simulink model "w2_warplab_trigger_proc"  (Simulink 7.7)
settings: Solver=ode45  StartTime=0.0  StopTime=1000  RelTol=1e-3
InitFcn:
  | w2_warplab_trigger_proc_init
StartFcn:
  | w2_warplab_trigger_proc_init
undefined symbols (not defined in the file or in its folder): gcbh, xlBlockLoadCallback, xlGetNormalizedPeriod
libraries: xbsIndex_r4 x819, simulink x1
(part 4 of 6)

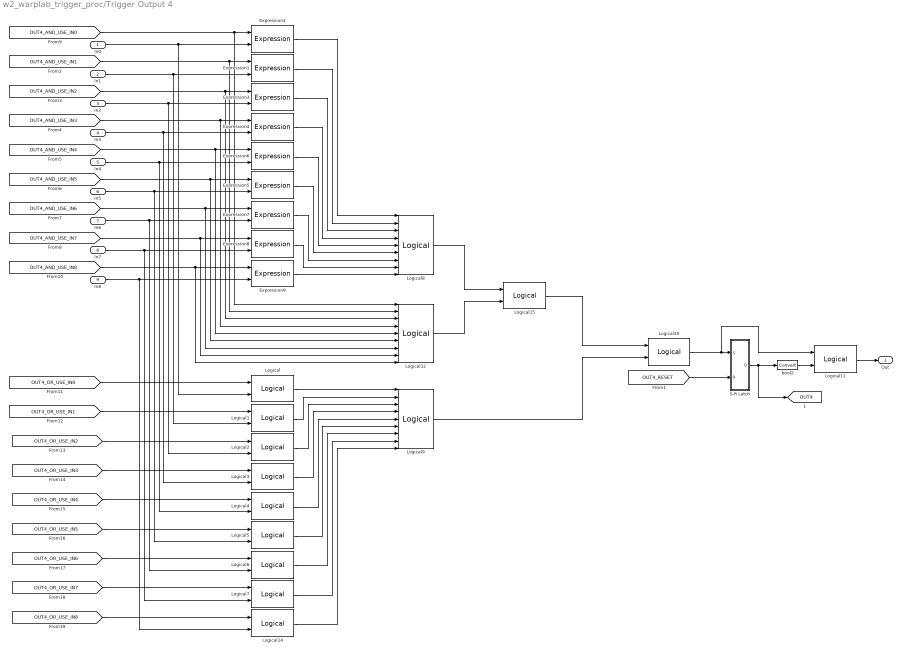
== system w2_warplab_trigger_proc/Trigger Output 4 ==
  In0 : Inport
  In1 : Inport  Port=2
  In2 : Inport  Port=3
  In3 : Inport  Port=4
  In4 : Inport  Port=5
  In5 : Inport  Port=6
  In6 : Inport  Port=7
  In7 : Inport  Port=8
  In8 : Inport  Port=9
  Expression{1..9} (9 alike) : xbsIndex_r4/Expression  expression=~a | (a & b)  align_bp=on  en=off  latency=0  precision=Full  arith_type=Unsigned  n_bits=16  bin_pt=0  dbl_ovrd=off  block_type=expr
  Logical{,1..7,14..15} (10 alike) : xbsIndex_r4/Logical  logical_function=AND  inputs=2  en=off  latency=0  precision=Full  arith_type=Unsigned  n_bits=16  bin_pt=0  align_bp=on  dbl_ovrd=off  block_type=logical
  Logical10 : xbsIndex_r4/Logical  logical_function=OR  inputs=2  en=off  latency=0  precision=Full  arith_type=Unsigned  n_bits=16  bin_pt=0  align_bp=on  dbl_ovrd=off  block_type=logical
  Logical11 : xbsIndex_r4/Logical  logical_function=OR  inputs=2  en=off  latency=0  precision=Full  arith_type=Unsigned  n_bits=16  bin_pt=0  align_bp=on  dbl_ovrd=off  block_type=logical
  Logical12 : xbsIndex_r4/Logical  logical_function=OR  inputs=9  en=off  latency=0  precision=Full  arith_type=Unsigned  n_bits=16  bin_pt=0  align_bp=on  dbl_ovrd=off  block_type=logical
  Logical8 : xbsIndex_r4/Logical  logical_function=AND  inputs=9  en=off  latency=0  precision=Full  arith_type=Unsigned  n_bits=16  bin_pt=0  align_bp=on  dbl_ovrd=off  block_type=logical
  Logical9 : xbsIndex_r4/Logical  logical_function=OR  inputs=9  en=off  latency=0  precision=Full  arith_type=Unsigned  n_bits=16  bin_pt=0  align_bp=on  dbl_ovrd=off  block_type=logical
  S-R Latch : Subsystem
  bool2 : xbsIndex_r4/Convert  gui_display_data_type=Boolean  arith_type=Boolean  n_bits=16  bin_pt=14  float_type=Single  exp_bits=8  fraction_bits=24  quantization=Truncate  overflow=Wrap  en=off  latency=0  dbl_ovrd=off  pipeline=off  block_type=convert
  Out : Outport
  tag scope: OUT4=global
  wires:
  [OUT4_AND_USE_IN0] -> Expression2/1, Logical12/1
  [OUT4_AND_USE_IN1] -> Expression1/1, Logical12/2
  [OUT4_AND_USE_IN2] -> Expression3/1, Logical12/3
  [OUT4_AND_USE_IN3] -> Expression4/1, Logical12/4
  [OUT4_AND_USE_IN4] -> Expression6/1, Logical12/5
  [OUT4_AND_USE_IN5] -> Expression5/1, Logical12/6
  [OUT4_AND_USE_IN6] -> Expression7/1, Logical12/7
  [OUT4_AND_USE_IN7] -> Expression8/1, Logical12/8
  In0/1 -> Logical/2, Expression2/2
  In1/1 -> Expression1/2, Logical1/2
  In2/1 -> Expression3/2, Logical2/2
  In3/1 -> Expression4/2, Logical3/2
  In4/1 -> Expression6/2, Logical4/2
  In5/1 -> Expression5/2, Logical5/2
  In6/1 -> Expression7/2, Logical6/2
  In7/1 -> Expression8/2, Logical7/2
  [OUT4_OR_USE_IN0] -> Logical/1
  [OUT4_OR_USE_IN1] -> Logical1/1
  Expression2/1 -> Logical8/1
  Expression1/1 -> Logical8/2
  Expression3/1 -> Logical8/3
  Expression4/1 -> Logical8/4
  Expression6/1 -> Logical8/5
  Expression5/1 -> Logical8/6
  Expression7/1 -> Logical8/7
  Expression8/1 -> Logical8/8
  Logical/1 -> Logical9/1
  Logical1/1 -> Logical9/2
  Logical2/1 -> Logical9/3
  Logical3/1 -> Logical9/4
  Logical4/1 -> Logical9/5
  Logical5/1 -> Logical9/6
  Logical6/1 -> Logical9/7
  Logical7/1 -> Logical9/8
  Logical9/1 -> Logical10/2
  Logical10/1 -> S-R Latch/1(S), Logical11/1
  [OUT4_RESET] -> S-R Latch/2(R)
  S-R Latch/1(Q) -> [OUT4], bool2/1
  Logical11/1 -> Out/1
  bool2/1 -> Logical11/2
  Logical12/1 -> Logical15/2
  Logical15/1 -> Logical10/1
  [OUT4_AND_USE_IN8] -> Expression9/1, Logical12/9
  In8/1 -> Expression9/2, Logical14/2
  Logical8/1 -> Logical15/1
  Expression9/1 -> Logical8/9
  [OUT4_OR_USE_IN2] -> Logical2/1
  [OUT4_OR_USE_IN3] -> Logical3/1
  [OUT4_OR_USE_IN4] -> Logical4/1
  [OUT4_OR_USE_IN5] -> Logical5/1
  [OUT4_OR_USE_IN6] -> Logical6/1
  [OUT4_OR_USE_IN7] -> Logical7/1
  [OUT4_OR_USE_IN8] -> Logical14/1
  Logical14/1 -> Logical9/9

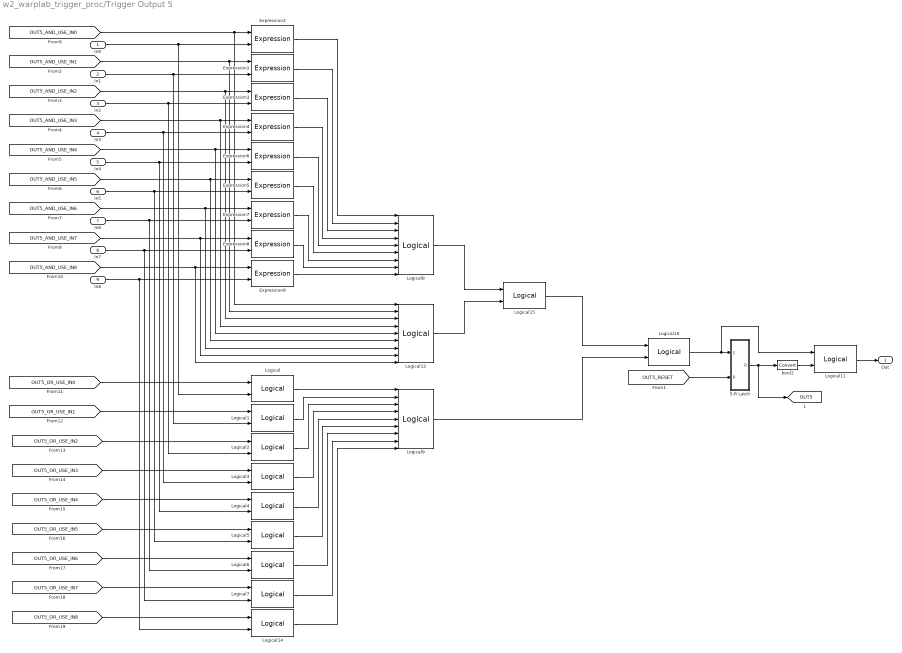
== system w2_warplab_trigger_proc/Trigger Output 5 ==
  In0 : Inport
  In1 : Inport  Port=2
  In2 : Inport  Port=3
  In3 : Inport  Port=4
  In4 : Inport  Port=5
  In5 : Inport  Port=6
  In6 : Inport  Port=7
  In7 : Inport  Port=8
  In8 : Inport  Port=9
  Expression{1..9} (9 alike) : xbsIndex_r4/Expression  expression=~a | (a & b)  align_bp=on  en=off  latency=0  precision=Full  arith_type=Unsigned  n_bits=16  bin_pt=0  dbl_ovrd=off  block_type=expr
  Logical{,1..7,14..15} (10 alike) : xbsIndex_r4/Logical  logical_function=AND  inputs=2  en=off  latency=0  precision=Full  arith_type=Unsigned  n_bits=16  bin_pt=0  align_bp=on  dbl_ovrd=off  block_type=logical
  Logical10 : xbsIndex_r4/Logical  logical_function=OR  inputs=2  en=off  latency=0  precision=Full  arith_type=Unsigned  n_bits=16  bin_pt=0  align_bp=on  dbl_ovrd=off  block_type=logical
  Logical11 : xbsIndex_r4/Logical  logical_function=OR  inputs=2  en=off  latency=0  precision=Full  arith_type=Unsigned  n_bits=16  bin_pt=0  align_bp=on  dbl_ovrd=off  block_type=logical
  Logical12 : xbsIndex_r4/Logical  logical_function=OR  inputs=9  en=off  latency=0  precision=Full  arith_type=Unsigned  n_bits=16  bin_pt=0  align_bp=on  dbl_ovrd=off  block_type=logical
  Logical8 : xbsIndex_r4/Logical  logical_function=AND  inputs=9  en=off  latency=0  precision=Full  arith_type=Unsigned  n_bits=16  bin_pt=0  align_bp=on  dbl_ovrd=off  block_type=logical
  Logical9 : xbsIndex_r4/Logical  logical_function=OR  inputs=9  en=off  latency=0  precision=Full  arith_type=Unsigned  n_bits=16  bin_pt=0  align_bp=on  dbl_ovrd=off  block_type=logical
  S-R Latch : Subsystem
  bool2 : xbsIndex_r4/Convert  gui_display_data_type=Boolean  arith_type=Boolean  n_bits=16  bin_pt=14  float_type=Single  exp_bits=8  fraction_bits=24  quantization=Truncate  overflow=Wrap  en=off  latency=0  dbl_ovrd=off  pipeline=off  block_type=convert
  Out : Outport
  tag scope: OUT5=global
  wires:
  [OUT5_AND_USE_IN0] -> Expression2/1, Logical12/1
  [OUT5_AND_USE_IN1] -> Expression1/1, Logical12/2
  [OUT5_AND_USE_IN2] -> Expression3/1, Logical12/3
  [OUT5_AND_USE_IN3] -> Expression4/1, Logical12/4
  [OUT5_AND_USE_IN4] -> Expression6/1, Logical12/5
  [OUT5_AND_USE_IN5] -> Expression5/1, Logical12/6
  [OUT5_AND_USE_IN6] -> Expression7/1, Logical12/7
  [OUT5_AND_USE_IN7] -> Expression8/1, Logical12/8
  In0/1 -> Logical/2, Expression2/2
  In1/1 -> Expression1/2, Logical1/2
  In2/1 -> Expression3/2, Logical2/2
  In3/1 -> Expression4/2, Logical3/2
  In4/1 -> Expression6/2, Logical4/2
  In5/1 -> Expression5/2, Logical5/2
  In6/1 -> Expression7/2, Logical6/2
  In7/1 -> Expression8/2, Logical7/2
  [OUT5_OR_USE_IN0] -> Logical/1
  [OUT5_OR_USE_IN1] -> Logical1/1
  Expression2/1 -> Logical8/1
  Expression1/1 -> Logical8/2
  Expression3/1 -> Logical8/3
  Expression4/1 -> Logical8/4
  Expression6/1 -> Logical8/5
  Expression5/1 -> Logical8/6
  Expression7/1 -> Logical8/7
  Expression8/1 -> Logical8/8
  Logical/1 -> Logical9/1
  Logical1/1 -> Logical9/2
  Logical2/1 -> Logical9/3
  Logical3/1 -> Logical9/4
  Logical4/1 -> Logical9/5
  Logical5/1 -> Logical9/6
  Logical6/1 -> Logical9/7
  Logical7/1 -> Logical9/8
  Logical9/1 -> Logical10/2
  Logical10/1 -> S-R Latch/1(S), Logical11/1
  [OUT5_RESET] -> S-R Latch/2(R)
  S-R Latch/1(Q) -> [OUT5], bool2/1
  Logical11/1 -> Out/1
  bool2/1 -> Logical11/2
  Logical12/1 -> Logical15/2
  Logical15/1 -> Logical10/1
  [OUT5_AND_USE_IN8] -> Expression9/1, Logical12/9
  In8/1 -> Expression9/2, Logical14/2
  Logical8/1 -> Logical15/1
  Expression9/1 -> Logical8/9
  [OUT5_OR_USE_IN2] -> Logical2/1
  [OUT5_OR_USE_IN3] -> Logical3/1
  [OUT5_OR_USE_IN4] -> Logical4/1
  [OUT5_OR_USE_IN5] -> Logical5/1
  [OUT5_OR_USE_IN6] -> Logical6/1
  [OUT5_OR_USE_IN7] -> Logical7/1
  [OUT5_OR_USE_IN8] -> Logical14/1
  Logical14/1 -> Logical9/9

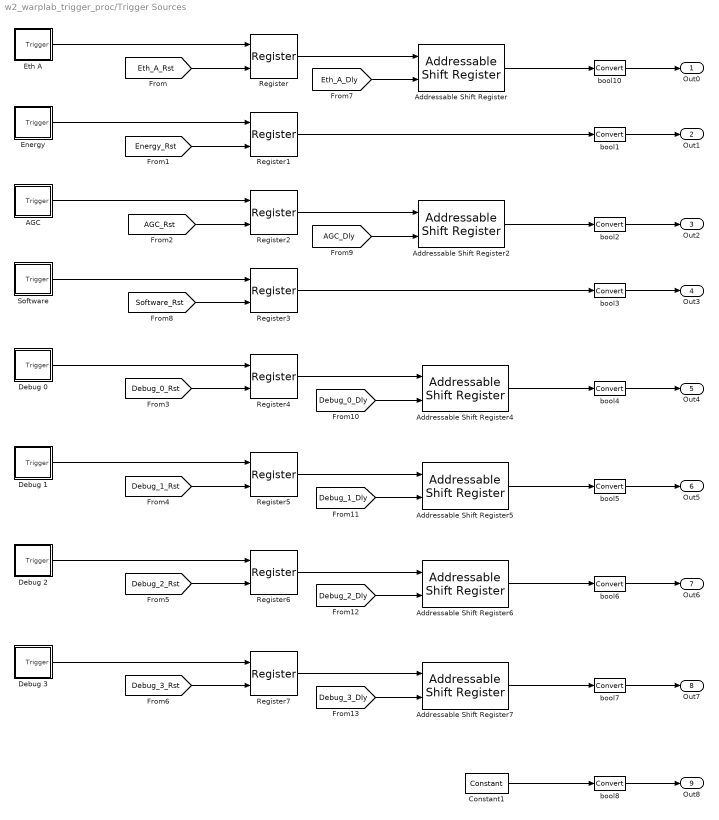
== system w2_warplab_trigger_proc/Trigger Sources ==
  AGC : Subsystem
  Addressable Shift Register{,2,4..7} (6 alike) : xbsIndex_r4/Addressable Shift Register  infer_latency=off  depth=32  initVector=[0]  en=off  dbl_ovrd=off  use_behavioral_HDL=off  Optimization=Resource  block_type=addrsr
      settings: infoedit="Delay of configurable length.  Any element in the delay line can be addressed and driven onto the output port.<br><br>Hardware notes: This block is implemented using SRL16s. If Virtex-4 or Spartan-3 device is used, multiple SRLC16s are cascaded together."
  Constant1 : xbsIndex_r4/Constant  const=0  gui_display_data_type=Fixed-point  arith_type=Unsigned  n_bits=1  bin_pt=0  preci_type=Single  exp_width=8  frac_width=24  explicit_period=off  period=1  equ=P=C  opselect=C  inp2=PCIN>>17  opr=+  inp1=P  carry=CIN  dbl_ovrd=off  block_type=constant
  Debug 0 : Subsystem
  Debug 1 : Subsystem
  Debug 2 : Subsystem
  Debug 3 : Subsystem
  Energy : Subsystem
  Eth A : Subsystem
  Register{,1..7} (8 alike) : xbsIndex_r4/Register  init=0  rst=on  en=off  dbl_ovrd=off  block_type=register
  Software : Subsystem
  bool{1..8,10} (9 alike) : xbsIndex_r4/Convert  gui_display_data_type=Boolean  arith_type=Boolean  n_bits=16  bin_pt=14  float_type=Single  exp_bits=8  fraction_bits=24  quantization=Truncate  overflow=Wrap  en=off  latency=0  dbl_ovrd=off  pipeline=off  block_type=convert
  Out0 : Outport
  Out1 : Outport  Port=2
  Out2 : Outport  Port=3
  Out3 : Outport  Port=4
  Out4 : Outport  Port=5
  Out5 : Outport  Port=6
  Out6 : Outport  Port=7
  Out7 : Outport  Port=8
  Out8 : Outport  Port=9
  wires:
  Energy/1(Trigger) -> Register1/1
  [Energy_Rst] -> Register1/2
  AGC/1(Trigger) -> Register2/1
  [AGC_Rst] -> Register2/2
  [Debug_0_Rst] -> Register4/2
  [Debug_1_Rst] -> Register5/2
  [Debug_2_Rst] -> Register6/2
  [Debug_3_Rst] -> Register7/2
  [Debug_0_Dly] -> Addressable Shift Register4/2
  Register4/1 -> Addressable Shift Register4/1
  [Debug_1_Dly] -> Addressable Shift Register5/2
  Register5/1 -> Addressable Shift Register5/1
  [Debug_2_Dly] -> Addressable Shift Register6/2
  Register6/1 -> Addressable Shift Register6/1
  [Debug_3_Dly] -> Addressable Shift Register7/2
  Register7/1 -> Addressable Shift Register7/1
  Software/1(Trigger) -> Register3/1
  [Software_Rst] -> Register3/2
  Register1/1 -> bool1/1
  Register3/1 -> bool3/1
  Addressable Shift Register4/1 -> bool4/1
  Addressable Shift Register5/1 -> bool5/1
  Addressable Shift Register6/1 -> bool6/1
  Addressable Shift Register7/1 -> bool7/1
  bool10/1 -> Out0/1
  bool1/1 -> Out1/1
  bool2/1 -> Out2/1
  bool3/1 -> Out3/1
  bool4/1 -> Out4/1
  bool5/1 -> Out5/1
  bool6/1 -> Out6/1
  bool7/1 -> Out7/1
  [AGC_Dly] -> Addressable Shift Register2/2
  Register2/1 -> Addressable Shift Register2/1
  Addressable Shift Register2/1 -> bool2/1
  bool8/1 -> Out8/1
  Debug 0/1(Trigger) -> Register4/1
  Debug 1/1(Trigger) -> Register5/1
  Debug 2/1(Trigger) -> Register6/1
  Debug 3/1(Trigger) -> Register7/1
  Constant1/1 -> bool8/1
  Eth A/1(Trigger) -> Register/1
  [Eth_A_Rst] -> Register/2
  Register/1 -> Addressable Shift Register/1
  [Eth_A_Dly] -> Addressable Shift Register/2
  Addressable Shift Register/1 -> bool10/1

== system w2_warplab_trigger_proc/Registers/Input Configuration Slice0 ==
  32b : Inport
  b29 : xbsIndex_r4/Slice  nbits=1  boolean_output=off  mode=Lower Bit Location + Width  bit1=0  base1=MSB of Input  bit0=29  base0=LSB of Input  dbl_ovrd=off  block_type=slice
  b30 : xbsIndex_r4/Slice  nbits=1  boolean_output=off  mode=Lower Bit Location + Width  bit1=0  base1=MSB of Input  bit0=30  base0=LSB of Input  dbl_ovrd=off  block_type=slice
  b31 : xbsIndex_r4/Slice  nbits=1  boolean_output=off  mode=Lower Bit Location + Width  bit1=0  base1=MSB of Input  bit0=31  base0=LSB of Input  dbl_ovrd=off  block_type=slice
  b[0:4] : xbsIndex_r4/Slice  nbits=5  boolean_output=off  mode=Lower Bit Location + Width  bit1=0  base1=MSB of Input  bit0=0  base0=LSB of Input  dbl_ovrd=off  block_type=slice
  Delay : Outport
  HW_SW_Sel : Outport  Port=2
  Debounce : Outport  Port=3
  Reset : Outport  Port=4
  wires:
  b31/1 -> Reset/1
  b30/1 -> Debounce/1
  b[0:4]/1 -> Delay/1
  32b/1 -> b[0:4]/1, b30/1, b31/1, b29/1
  b29/1 -> HW_SW_Sel/1

== system w2_warplab_trigger_proc/Registers/Input Configuration Slice1 ==
  32b : Inport
  b30 : xbsIndex_r4/Slice  nbits=1  boolean_output=off  mode=Lower Bit Location + Width  bit1=0  base1=MSB of Input  bit0=30  base0=LSB of Input  dbl_ovrd=off  block_type=slice
  b31 : xbsIndex_r4/Slice  nbits=1  boolean_output=off  mode=Lower Bit Location + Width  bit1=0  base1=MSB of Input  bit0=31  base0=LSB of Input  dbl_ovrd=off  block_type=slice
  b[0:4] : xbsIndex_r4/Slice  nbits=5  boolean_output=off  mode=Lower Bit Location + Width  bit1=0  base1=MSB of Input  bit0=0  base0=LSB of Input  dbl_ovrd=off  block_type=slice
  Delay : Outport
  Debounce : Outport  Port=2
  Reset : Outport  Port=3
  wires:
  b31/1 -> Reset/1
  b30/1 -> Debounce/1
  b[0:4]/1 -> Delay/1
  32b/1 -> b[0:4]/1, b30/1, b31/1

== system w2_warplab_trigger_proc/Registers/Input Configuration Slice2 ==
  32b : Inport
  b30 : xbsIndex_r4/Slice  nbits=1  boolean_output=off  mode=Lower Bit Location + Width  bit1=0  base1=MSB of Input  bit0=30  base0=LSB of Input  dbl_ovrd=off  block_type=slice
  b31 : xbsIndex_r4/Slice  nbits=1  boolean_output=off  mode=Lower Bit Location + Width  bit1=0  base1=MSB of Input  bit0=31  base0=LSB of Input  dbl_ovrd=off  block_type=slice
  b[0:4] : xbsIndex_r4/Slice  nbits=5  boolean_output=off  mode=Lower Bit Location + Width  bit1=0  base1=MSB of Input  bit0=0  base0=LSB of Input  dbl_ovrd=off  block_type=slice
  Delay : Outport
  Debounce : Outport  Port=2
  Reset : Outport  Port=3
  wires:
  b31/1 -> Reset/1
  b30/1 -> Debounce/1
  b[0:4]/1 -> Delay/1
  32b/1 -> b[0:4]/1, b30/1, b31/1

== system w2_warplab_trigger_proc/Registers/Input Configuration Slice3 ==
  32b : Inport
  b30 : xbsIndex_r4/Slice  nbits=1  boolean_output=off  mode=Lower Bit Location + Width  bit1=0  base1=MSB of Input  bit0=30  base0=LSB of Input  dbl_ovrd=off  block_type=slice
  b31 : xbsIndex_r4/Slice  nbits=1  boolean_output=off  mode=Lower Bit Location + Width  bit1=0  base1=MSB of Input  bit0=31  base0=LSB of Input  dbl_ovrd=off  block_type=slice
  b[0:4] : xbsIndex_r4/Slice  nbits=5  boolean_output=off  mode=Lower Bit Location + Width  bit1=0  base1=MSB of Input  bit0=0  base0=LSB of Input  dbl_ovrd=off  block_type=slice
  Delay : Outport
  Debounce : Outport  Port=2
  Reset : Outport  Port=3
  wires:
  b31/1 -> Reset/1
  b30/1 -> Debounce/1
  b[0:4]/1 -> Delay/1
  32b/1 -> b[0:4]/1, b30/1, b31/1

== system w2_warplab_trigger_proc/Registers/Input Configuration Slice4 ==
  32b : Inport
  b30 : xbsIndex_r4/Slice  nbits=1  boolean_output=off  mode=Lower Bit Location + Width  bit1=0  base1=MSB of Input  bit0=30  base0=LSB of Input  dbl_ovrd=off  block_type=slice
  b31 : xbsIndex_r4/Slice  nbits=1  boolean_output=off  mode=Lower Bit Location + Width  bit1=0  base1=MSB of Input  bit0=31  base0=LSB of Input  dbl_ovrd=off  block_type=slice
  b[0:4] : xbsIndex_r4/Slice  nbits=5  boolean_output=off  mode=Lower Bit Location + Width  bit1=0  base1=MSB of Input  bit0=0  base0=LSB of Input  dbl_ovrd=off  block_type=slice
  Delay : Outport
  Debounce : Outport  Port=2
  Reset : Outport  Port=3
  wires:
  b31/1 -> Reset/1
  b30/1 -> Debounce/1
  b[0:4]/1 -> Delay/1
  32b/1 -> b[0:4]/1, b30/1, b31/1

== system w2_warplab_trigger_proc/Registers/Input Configuration Slice5 ==
  32b : Inport
  b30 : xbsIndex_r4/Slice  nbits=1  boolean_output=off  mode=Lower Bit Location + Width  bit1=0  base1=MSB of Input  bit0=30  base0=LSB of Input  dbl_ovrd=off  block_type=slice
  b31 : xbsIndex_r4/Slice  nbits=1  boolean_output=off  mode=Lower Bit Location + Width  bit1=0  base1=MSB of Input  bit0=31  base0=LSB of Input  dbl_ovrd=off  block_type=slice
  b[0:4] : xbsIndex_r4/Slice  nbits=5  boolean_output=off  mode=Lower Bit Location + Width  bit1=0  base1=MSB of Input  bit0=0  base0=LSB of Input  dbl_ovrd=off  block_type=slice
  Delay : Outport
  Debounce : Outport  Port=2
  Reset : Outport  Port=3
  wires:
  b31/1 -> Reset/1
  b30/1 -> Debounce/1
  b[0:4]/1 -> Delay/1
  32b/1 -> b[0:4]/1, b30/1, b31/1

== system w2_warplab_trigger_proc/Registers/Input Configuration Slice6 ==
  32b : Inport
  b30 : xbsIndex_r4/Slice  nbits=1  boolean_output=off  mode=Lower Bit Location + Width  bit1=0  base1=MSB of Input  bit0=30  base0=LSB of Input  dbl_ovrd=off  block_type=slice
  b31 : xbsIndex_r4/Slice  nbits=1  boolean_output=off  mode=Lower Bit Location + Width  bit1=0  base1=MSB of Input  bit0=31  base0=LSB of Input  dbl_ovrd=off  block_type=slice
  b[0:4] : xbsIndex_r4/Slice  nbits=5  boolean_output=off  mode=Lower Bit Location + Width  bit1=0  base1=MSB of Input  bit0=0  base0=LSB of Input  dbl_ovrd=off  block_type=slice
  Delay : Outport
  Debounce : Outport  Port=2
  Reset : Outport  Port=3
  wires:
  b31/1 -> Reset/1
  b30/1 -> Debounce/1
  b[0:4]/1 -> Delay/1
  32b/1 -> b[0:4]/1, b30/1, b31/1

== system w2_warplab_trigger_proc/Registers/Input Configuration Slice7 ==
  32b : Inport
  b30 : xbsIndex_r4/Slice  nbits=1  boolean_output=off  mode=Lower Bit Location + Width  bit1=0  base1=MSB of Input  bit0=30  base0=LSB of Input  dbl_ovrd=off  block_type=slice
  b31 : xbsIndex_r4/Slice  nbits=1  boolean_output=off  mode=Lower Bit Location + Width  bit1=0  base1=MSB of Input  bit0=31  base0=LSB of Input  dbl_ovrd=off  block_type=slice
  b[0:4] : xbsIndex_r4/Slice  nbits=5  boolean_output=off  mode=Lower Bit Location + Width  bit1=0  base1=MSB of Input  bit0=0  base0=LSB of Input  dbl_ovrd=off  block_type=slice
  Delay : Outport
  Debounce : Outport  Port=2
  Reset : Outport  Port=3
  wires:
  b31/1 -> Reset/1
  b30/1 -> Debounce/1
  b[0:4]/1 -> Delay/1
  32b/1 -> b[0:4]/1, b30/1, b31/1

== system w2_warplab_trigger_proc/Registers/Input Configuration Slice8 ==
  32b : Inport
  b29 : xbsIndex_r4/Slice  nbits=1  boolean_output=off  mode=Lower Bit Location + Width  bit1=0  base1=MSB of Input  bit0=29  base0=LSB of Input  dbl_ovrd=off  block_type=slice
  b30 : xbsIndex_r4/Slice  nbits=1  boolean_output=off  mode=Lower Bit Location + Width  bit1=0  base1=MSB of Input  bit0=30  base0=LSB of Input  dbl_ovrd=off  block_type=slice
  b31 : xbsIndex_r4/Slice  nbits=1  boolean_output=off  mode=Lower Bit Location + Width  bit1=0  base1=MSB of Input  bit0=31  base0=LSB of Input  dbl_ovrd=off  block_type=slice
  b[0:4] : xbsIndex_r4/Slice  nbits=5  boolean_output=off  mode=Lower Bit Location + Width  bit1=0  base1=MSB of Input  bit0=0  base0=LSB of Input  dbl_ovrd=off  block_type=slice
  Delay : Outport
  HW_SW_Sel : Outport  Port=2
  Debounce : Outport  Port=3
  Reset : Outport  Port=4
  wires:
  b31/1 -> Reset/1
  b30/1 -> Debounce/1
  b[0:4]/1 -> Delay/1
  32b/1 -> b[0:4]/1, b30/1, b31/1, b29/1
  b29/1 -> HW_SW_Sel/1

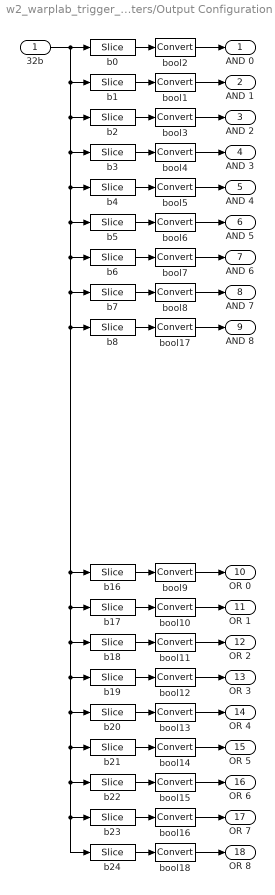
== system w2_warplab_trigger_proc/Registers/Output Configuration Slice ==
  32b : Inport
  b0 : xbsIndex_r4/Slice  nbits=1  boolean_output=off  mode=Lower Bit Location + Width  bit1=0  base1=MSB of Input  bit0=0  base0=LSB of Input  dbl_ovrd=off  block_type=slice
  b1 : xbsIndex_r4/Slice  nbits=1  boolean_output=off  mode=Lower Bit Location + Width  bit1=0  base1=MSB of Input  bit0=1  base0=LSB of Input  dbl_ovrd=off  block_type=slice
  b16 : xbsIndex_r4/Slice  nbits=1  boolean_output=off  mode=Lower Bit Location + Width  bit1=0  base1=MSB of Input  bit0=16  base0=LSB of Input  dbl_ovrd=off  block_type=slice
  b17 : xbsIndex_r4/Slice  nbits=1  boolean_output=off  mode=Lower Bit Location + Width  bit1=0  base1=MSB of Input  bit0=17  base0=LSB of Input  dbl_ovrd=off  block_type=slice
  b18 : xbsIndex_r4/Slice  nbits=1  boolean_output=off  mode=Lower Bit Location + Width  bit1=0  base1=MSB of Input  bit0=18  base0=LSB of Input  dbl_ovrd=off  block_type=slice
  b19 : xbsIndex_r4/Slice  nbits=1  boolean_output=off  mode=Lower Bit Location + Width  bit1=0  base1=MSB of Input  bit0=19  base0=LSB of Input  dbl_ovrd=off  block_type=slice
  b2 : xbsIndex_r4/Slice  nbits=1  boolean_output=off  mode=Lower Bit Location + Width  bit1=0  base1=MSB of Input  bit0=2  base0=LSB of Input  dbl_ovrd=off  block_type=slice
  b20 : xbsIndex_r4/Slice  nbits=1  boolean_output=off  mode=Lower Bit Location + Width  bit1=0  base1=MSB of Input  bit0=20  base0=LSB of Input  dbl_ovrd=off  block_type=slice
  b21 : xbsIndex_r4/Slice  nbits=1  boolean_output=off  mode=Lower Bit Location + Width  bit1=0  base1=MSB of Input  bit0=21  base0=LSB of Input  dbl_ovrd=off  block_type=slice
  b22 : xbsIndex_r4/Slice  nbits=1  boolean_output=off  mode=Lower Bit Location + Width  bit1=0  base1=MSB of Input  bit0=22  base0=LSB of Input  dbl_ovrd=off  block_type=slice
  b23 : xbsIndex_r4/Slice  nbits=1  boolean_output=off  mode=Lower Bit Location + Width  bit1=0  base1=MSB of Input  bit0=23  base0=LSB of Input  dbl_ovrd=off  block_type=slice
  b24 : xbsIndex_r4/Slice  nbits=1  boolean_output=off  mode=Lower Bit Location + Width  bit1=0  base1=MSB of Input  bit0=24  base0=LSB of Input  dbl_ovrd=off  block_type=slice
  b3 : xbsIndex_r4/Slice  nbits=1  boolean_output=off  mode=Lower Bit Location + Width  bit1=0  base1=MSB of Input  bit0=3  base0=LSB of Input  dbl_ovrd=off  block_type=slice
  b4 : xbsIndex_r4/Slice  nbits=1  boolean_output=off  mode=Lower Bit Location + Width  bit1=0  base1=MSB of Input  bit0=4  base0=LSB of Input  dbl_ovrd=off  block_type=slice
  b5 : xbsIndex_r4/Slice  nbits=1  boolean_output=off  mode=Lower Bit Location + Width  bit1=0  base1=MSB of Input  bit0=5  base0=LSB of Input  dbl_ovrd=off  block_type=slice
  b6 : xbsIndex_r4/Slice  nbits=1  boolean_output=off  mode=Lower Bit Location + Width  bit1=0  base1=MSB of Input  bit0=6  base0=LSB of Input  dbl_ovrd=off  block_type=slice
  b7 : xbsIndex_r4/Slice  nbits=1  boolean_output=off  mode=Lower Bit Location + Width  bit1=0  base1=MSB of Input  bit0=7  base0=LSB of Input  dbl_ovrd=off  block_type=slice
  b8 : xbsIndex_r4/Slice  nbits=1  boolean_output=off  mode=Lower Bit Location + Width  bit1=0  base1=MSB of Input  bit0=8  base0=LSB of Input  dbl_ovrd=off  block_type=slice
  bool{1..18} (18 alike) : xbsIndex_r4/Convert  gui_display_data_type=Boolean  arith_type=Boolean  n_bits=16  bin_pt=14  float_type=Single  exp_bits=8  fraction_bits=24  quantization=Truncate  overflow=Wrap  en=off  latency=0  dbl_ovrd=off  pipeline=off  block_type=convert
  AND 0 : Outport
  AND 1 : Outport  Port=2
  AND 2 : Outport  Port=3
  AND 3 : Outport  Port=4
  AND 4 : Outport  Port=5
  AND 5 : Outport  Port=6
  AND 6 : Outport  Port=7
  AND 7 : Outport  Port=8
  AND 8 : Outport  Port=9
  OR 0 : Outport  Port=10
  OR 1 : Outport  Port=11
  OR 2 : Outport  Port=12
  OR 3 : Outport  Port=13
  OR 4 : Outport  Port=14
  OR 5 : Outport  Port=15
  OR 6 : Outport  Port=16
  OR 7 : Outport  Port=17
  OR 8 : Outport  Port=18
  wires:
  32b/1 -> b0/1, b1/1, b2/1, b3/1, b4/1, b5/1, b6/1, b7/1, b16/1, b17/1, b18/1, b19/1, b20/1, b21/1, b22/1, b23/1, b24/1, b8/1
  b0/1 -> bool2/1
  b1/1 -> bool1/1
  b2/1 -> bool3/1
  b3/1 -> bool4/1
  b4/1 -> bool5/1
  b5/1 -> bool6/1
  b6/1 -> bool7/1
  b7/1 -> bool8/1
  b16/1 -> bool9/1
  b17/1 -> bool10/1
  b18/1 -> bool11/1
  b19/1 -> bool12/1
  b20/1 -> bool13/1
  b21/1 -> bool14/1
  b22/1 -> bool15/1
  b23/1 -> bool16/1
  bool2/1 -> AND 0/1
  bool1/1 -> AND 1/1
  bool3/1 -> AND 2/1
  bool4/1 -> AND 3/1
  bool5/1 -> AND 4/1
  bool6/1 -> AND 5/1
  bool7/1 -> AND 6/1
  bool8/1 -> AND 7/1
  bool9/1 -> OR 0/1
  bool10/1 -> OR 1/1
  bool11/1 -> OR 2/1
  bool12/1 -> OR 3/1
  bool13/1 -> OR 4/1
  bool14/1 -> OR 5/1
  bool15/1 -> OR 6/1
  bool16/1 -> OR 7/1
  b8/1 -> bool17/1
  bool17/1 -> AND 8/1
  b24/1 -> bool18/1
  bool18/1 -> OR 8/1

== system w2_warplab_trigger_proc/Registers/Output Configuration Slice1 ==
  32b : Inport
  (LSB+0):(LSB+4) : xbsIndex_r4/Slice  nbits=5  boolean_output=off  mode=Lower Bit Location + Width  bit1=0  base1=MSB of Input  bit0=0  base0=LSB of Input  dbl_ovrd=off  block_type=slice
  b31 : xbsIndex_r4/Slice  nbits=1  boolean_output=off  mode=Lower Bit Location + Width  bit1=0  base1=MSB of Input  bit0=31  base0=LSB of Input  dbl_ovrd=off  block_type=slice
  bool17 : xbsIndex_r4/Convert  gui_display_data_type=Boolean  arith_type=Boolean  n_bits=16  bin_pt=14  float_type=Single  exp_bits=8  fraction_bits=24  quantization=Truncate  overflow=Wrap  en=off  latency=0  dbl_ovrd=off  pipeline=off  block_type=convert
  DLY : Outport
  RESET : Outport  Port=2
  wires:
  32b/1 -> b31/1, (LSB+0):(LSB+4)/1
  b31/1 -> bool17/1
  bool17/1 -> RESET/1
  (LSB+0):(LSB+4)/1 -> DLY/1

== system w2_warplab_trigger_proc/Registers/Output Configuration Slice10 ==
  32b : Inport
  b16 : xbsIndex_r4/Slice  nbits=5  boolean_output=off  mode=Lower Bit Location + Width  bit1=0  base1=MSB of Input  bit0=0  base0=LSB of Input  dbl_ovrd=off  block_type=slice
  b31 : xbsIndex_r4/Slice  nbits=1  boolean_output=off  mode=Lower Bit Location + Width  bit1=0  base1=MSB of Input  bit0=31  base0=LSB of Input  dbl_ovrd=off  block_type=slice
  bool17 : xbsIndex_r4/Convert  gui_display_data_type=Boolean  arith_type=Boolean  n_bits=16  bin_pt=14  float_type=Single  exp_bits=8  fraction_bits=24  quantization=Truncate  overflow=Wrap  en=off  latency=0  dbl_ovrd=off  pipeline=off  block_type=convert
  DLY : Outport
  RESET : Outport  Port=2
  wires:
  32b/1 -> b31/1, b16/1
  b31/1 -> bool17/1
  bool17/1 -> RESET/1
  b16/1 -> DLY/1

== system w2_warplab_trigger_proc/Registers/Output Configuration Slice11 ==
  32b : Inport
  b16 : xbsIndex_r4/Slice  nbits=5  boolean_output=off  mode=Lower Bit Location + Width  bit1=0  base1=MSB of Input  bit0=0  base0=LSB of Input  dbl_ovrd=off  block_type=slice
  b31 : xbsIndex_r4/Slice  nbits=1  boolean_output=off  mode=Lower Bit Location + Width  bit1=0  base1=MSB of Input  bit0=31  base0=LSB of Input  dbl_ovrd=off  block_type=slice
  bool17 : xbsIndex_r4/Convert  gui_display_data_type=Boolean  arith_type=Boolean  n_bits=16  bin_pt=14  float_type=Single  exp_bits=8  fraction_bits=24  quantization=Truncate  overflow=Wrap  en=off  latency=0  dbl_ovrd=off  pipeline=off  block_type=convert
  DLY : Outport
  RESET : Outport  Port=2
  wires:
  32b/1 -> b31/1, b16/1
  b31/1 -> bool17/1
  bool17/1 -> RESET/1
  b16/1 -> DLY/1

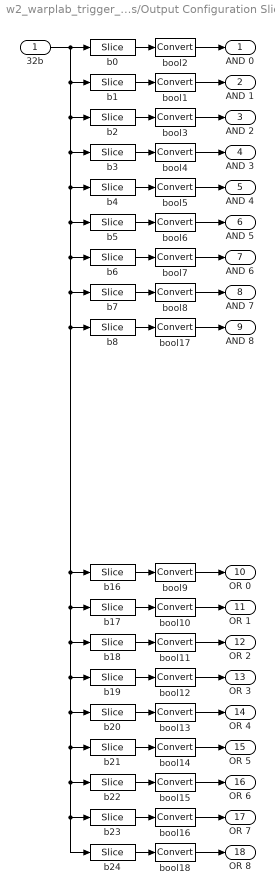
== system w2_warplab_trigger_proc/Registers/Output Configuration Slice12 ==
  32b : Inport
  b0 : xbsIndex_r4/Slice  nbits=1  boolean_output=off  mode=Lower Bit Location + Width  bit1=0  base1=MSB of Input  bit0=0  base0=LSB of Input  dbl_ovrd=off  block_type=slice
  b1 : xbsIndex_r4/Slice  nbits=1  boolean_output=off  mode=Lower Bit Location + Width  bit1=0  base1=MSB of Input  bit0=1  base0=LSB of Input  dbl_ovrd=off  block_type=slice
  b16 : xbsIndex_r4/Slice  nbits=1  boolean_output=off  mode=Lower Bit Location + Width  bit1=0  base1=MSB of Input  bit0=16  base0=LSB of Input  dbl_ovrd=off  block_type=slice
  b17 : xbsIndex_r4/Slice  nbits=1  boolean_output=off  mode=Lower Bit Location + Width  bit1=0  base1=MSB of Input  bit0=17  base0=LSB of Input  dbl_ovrd=off  block_type=slice
  b18 : xbsIndex_r4/Slice  nbits=1  boolean_output=off  mode=Lower Bit Location + Width  bit1=0  base1=MSB of Input  bit0=18  base0=LSB of Input  dbl_ovrd=off  block_type=slice
  b19 : xbsIndex_r4/Slice  nbits=1  boolean_output=off  mode=Lower Bit Location + Width  bit1=0  base1=MSB of Input  bit0=19  base0=LSB of Input  dbl_ovrd=off  block_type=slice
  b2 : xbsIndex_r4/Slice  nbits=1  boolean_output=off  mode=Lower Bit Location + Width  bit1=0  base1=MSB of Input  bit0=2  base0=LSB of Input  dbl_ovrd=off  block_type=slice
  b20 : xbsIndex_r4/Slice  nbits=1  boolean_output=off  mode=Lower Bit Location + Width  bit1=0  base1=MSB of Input  bit0=20  base0=LSB of Input  dbl_ovrd=off  block_type=slice
  b21 : xbsIndex_r4/Slice  nbits=1  boolean_output=off  mode=Lower Bit Location + Width  bit1=0  base1=MSB of Input  bit0=21  base0=LSB of Input  dbl_ovrd=off  block_type=slice
  b22 : xbsIndex_r4/Slice  nbits=1  boolean_output=off  mode=Lower Bit Location + Width  bit1=0  base1=MSB of Input  bit0=22  base0=LSB of Input  dbl_ovrd=off  block_type=slice
  b23 : xbsIndex_r4/Slice  nbits=1  boolean_output=off  mode=Lower Bit Location + Width  bit1=0  base1=MSB of Input  bit0=23  base0=LSB of Input  dbl_ovrd=off  block_type=slice
  b24 : xbsIndex_r4/Slice  nbits=1  boolean_output=off  mode=Lower Bit Location + Width  bit1=0  base1=MSB of Input  bit0=24  base0=LSB of Input  dbl_ovrd=off  block_type=slice
  b3 : xbsIndex_r4/Slice  nbits=1  boolean_output=off  mode=Lower Bit Location + Width  bit1=0  base1=MSB of Input  bit0=3  base0=LSB of Input  dbl_ovrd=off  block_type=slice
  b4 : xbsIndex_r4/Slice  nbits=1  boolean_output=off  mode=Lower Bit Location + Width  bit1=0  base1=MSB of Input  bit0=4  base0=LSB of Input  dbl_ovrd=off  block_type=slice
  b5 : xbsIndex_r4/Slice  nbits=1  boolean_output=off  mode=Lower Bit Location + Width  bit1=0  base1=MSB of Input  bit0=5  base0=LSB of Input  dbl_ovrd=off  block_type=slice
  b6 : xbsIndex_r4/Slice  nbits=1  boolean_output=off  mode=Lower Bit Location + Width  bit1=0  base1=MSB of Input  bit0=6  base0=LSB of Input  dbl_ovrd=off  block_type=slice
  b7 : xbsIndex_r4/Slice  nbits=1  boolean_output=off  mode=Lower Bit Location + Width  bit1=0  base1=MSB of Input  bit0=7  base0=LSB of Input  dbl_ovrd=off  block_type=slice
  b8 : xbsIndex_r4/Slice  nbits=1  boolean_output=off  mode=Lower Bit Location + Width  bit1=0  base1=MSB of Input  bit0=8  base0=LSB of Input  dbl_ovrd=off  block_type=slice
  bool{1..18} (18 alike) : xbsIndex_r4/Convert  gui_display_data_type=Boolean  arith_type=Boolean  n_bits=16  bin_pt=14  float_type=Single  exp_bits=8  fraction_bits=24  quantization=Truncate  overflow=Wrap  en=off  latency=0  dbl_ovrd=off  pipeline=off  block_type=convert
  AND 0 : Outport
  AND 1 : Outport  Port=2
  AND 2 : Outport  Port=3
  AND 3 : Outport  Port=4
  AND 4 : Outport  Port=5
  AND 5 : Outport  Port=6
  AND 6 : Outport  Port=7
  AND 7 : Outport  Port=8
  AND 8 : Outport  Port=9
  OR 0 : Outport  Port=10
  OR 1 : Outport  Port=11
  OR 2 : Outport  Port=12
  OR 3 : Outport  Port=13
  OR 4 : Outport  Port=14
  OR 5 : Outport  Port=15
  OR 6 : Outport  Port=16
  OR 7 : Outport  Port=17
  OR 8 : Outport  Port=18
  wires:
  32b/1 -> b0/1, b1/1, b2/1, b3/1, b4/1, b5/1, b6/1, b7/1, b16/1, b17/1, b18/1, b19/1, b20/1, b21/1, b22/1, b23/1, b24/1, b8/1
  b0/1 -> bool2/1
  b1/1 -> bool1/1
  b2/1 -> bool3/1
  b3/1 -> bool4/1
  b4/1 -> bool5/1
  b5/1 -> bool6/1
  b6/1 -> bool7/1
  b7/1 -> bool8/1
  b16/1 -> bool9/1
  b17/1 -> bool10/1
  b18/1 -> bool11/1
  b19/1 -> bool12/1
  b20/1 -> bool13/1
  b21/1 -> bool14/1
  b22/1 -> bool15/1
  b23/1 -> bool16/1
  bool2/1 -> AND 0/1
  bool1/1 -> AND 1/1
  bool3/1 -> AND 2/1
  bool4/1 -> AND 3/1
  bool5/1 -> AND 4/1
  bool6/1 -> AND 5/1
  bool7/1 -> AND 6/1
  bool8/1 -> AND 7/1
  bool9/1 -> OR 0/1
  bool10/1 -> OR 1/1
  bool11/1 -> OR 2/1
  bool12/1 -> OR 3/1
  bool13/1 -> OR 4/1
  bool14/1 -> OR 5/1
  bool15/1 -> OR 6/1
  bool16/1 -> OR 7/1
  b8/1 -> bool17/1
  bool17/1 -> AND 8/1
  b24/1 -> bool18/1
  bool18/1 -> OR 8/1

== system w2_warplab_trigger_proc/Registers/Output Configuration Slice13 ==
  32b : Inport
  b16 : xbsIndex_r4/Slice  nbits=5  boolean_output=off  mode=Lower Bit Location + Width  bit1=0  base1=MSB of Input  bit0=0  base0=LSB of Input  dbl_ovrd=off  block_type=slice
  b31 : xbsIndex_r4/Slice  nbits=1  boolean_output=off  mode=Lower Bit Location + Width  bit1=0  base1=MSB of Input  bit0=31  base0=LSB of Input  dbl_ovrd=off  block_type=slice
  bool17 : xbsIndex_r4/Convert  gui_display_data_type=Boolean  arith_type=Boolean  n_bits=16  bin_pt=14  float_type=Single  exp_bits=8  fraction_bits=24  quantization=Truncate  overflow=Wrap  en=off  latency=0  dbl_ovrd=off  pipeline=off  block_type=convert
  DLY : Outport
  RESET : Outport  Port=2
  wires:
  32b/1 -> b31/1, b16/1
  b31/1 -> bool17/1
  bool17/1 -> RESET/1
  b16/1 -> DLY/1

== system w2_warplab_trigger_proc/Registers/Output Configuration Slice14 ==
  32b : Inport
  b0 : xbsIndex_r4/Slice  nbits=1  boolean_output=off  mode=Lower Bit Location + Width  bit1=0  base1=MSB of Input  bit0=0  base0=LSB of Input  dbl_ovrd=off  block_type=slice
  b1 : xbsIndex_r4/Slice  nbits=1  boolean_output=off  mode=Lower Bit Location + Width  bit1=0  base1=MSB of Input  bit0=1  base0=LSB of Input  dbl_ovrd=off  block_type=slice
  b16 : xbsIndex_r4/Slice  nbits=1  boolean_output=off  mode=Lower Bit Location + Width  bit1=0  base1=MSB of Input  bit0=16  base0=LSB of Input  dbl_ovrd=off  block_type=slice
  b17 : xbsIndex_r4/Slice  nbits=1  boolean_output=off  mode=Lower Bit Location + Width  bit1=0  base1=MSB of Input  bit0=17  base0=LSB of Input  dbl_ovrd=off  block_type=slice
  b18 : xbsIndex_r4/Slice  nbits=1  boolean_output=off  mode=Lower Bit Location + Width  bit1=0  base1=MSB of Input  bit0=18  base0=LSB of Input  dbl_ovrd=off  block_type=slice
  b19 : xbsIndex_r4/Slice  nbits=1  boolean_output=off  mode=Lower Bit Location + Width  bit1=0  base1=MSB of Input  bit0=19  base0=LSB of Input  dbl_ovrd=off  block_type=slice
  b2 : xbsIndex_r4/Slice  nbits=1  boolean_output=off  mode=Lower Bit Location + Width  bit1=0  base1=MSB of Input  bit0=2  base0=LSB of Input  dbl_ovrd=off  block_type=slice
  b20 : xbsIndex_r4/Slice  nbits=1  boolean_output=off  mode=Lower Bit Location + Width  bit1=0  base1=MSB of Input  bit0=20  base0=LSB of Input  dbl_ovrd=off  block_type=slice
  b21 : xbsIndex_r4/Slice  nbits=1  boolean_output=off  mode=Lower Bit Location + Width  bit1=0  base1=MSB of Input  bit0=21  base0=LSB of Input  dbl_ovrd=off  block_type=slice
  b22 : xbsIndex_r4/Slice  nbits=1  boolean_output=off  mode=Lower Bit Location + Width  bit1=0  base1=MSB of Input  bit0=22  base0=LSB of Input  dbl_ovrd=off  block_type=slice
  b23 : xbsIndex_r4/Slice  nbits=1  boolean_output=off  mode=Lower Bit Location + Width  bit1=0  base1=MSB of Input  bit0=23  base0=LSB of Input  dbl_ovrd=off  block_type=slice
  b24 : xbsIndex_r4/Slice  nbits=1  boolean_output=off  mode=Lower Bit Location + Width  bit1=0  base1=MSB of Input  bit0=24  base0=LSB of Input  dbl_ovrd=off  block_type=slice
  b3 : xbsIndex_r4/Slice  nbits=1  boolean_output=off  mode=Lower Bit Location + Width  bit1=0  base1=MSB of Input  bit0=3  base0=LSB of Input  dbl_ovrd=off  block_type=slice
  b4 : xbsIndex_r4/Slice  nbits=1  boolean_output=off  mode=Lower Bit Location + Width  bit1=0  base1=MSB of Input  bit0=4  base0=LSB of Input  dbl_ovrd=off  block_type=slice
  b5 : xbsIndex_r4/Slice  nbits=1  boolean_output=off  mode=Lower Bit Location + Width  bit1=0  base1=MSB of Input  bit0=5  base0=LSB of Input  dbl_ovrd=off  block_type=slice
  b6 : xbsIndex_r4/Slice  nbits=1  boolean_output=off  mode=Lower Bit Location + Width  bit1=0  base1=MSB of Input  bit0=6  base0=LSB of Input  dbl_ovrd=off  block_type=slice
  b7 : xbsIndex_r4/Slice  nbits=1  boolean_output=off  mode=Lower Bit Location + Width  bit1=0  base1=MSB of Input  bit0=7  base0=LSB of Input  dbl_ovrd=off  block_type=slice
  b8 : xbsIndex_r4/Slice  nbits=1  boolean_output=off  mode=Lower Bit Location + Width  bit1=0  base1=MSB of Input  bit0=8  base0=LSB of Input  dbl_ovrd=off  block_type=slice
  bool{1..18} (18 alike) : xbsIndex_r4/Convert  gui_display_data_type=Boolean  arith_type=Boolean  n_bits=16  bin_pt=14  float_type=Single  exp_bits=8  fraction_bits=24  quantization=Truncate  overflow=Wrap  en=off  latency=0  dbl_ovrd=off  pipeline=off  block_type=convert
  AND 0 : Outport
  AND 1 : Outport  Port=2
  AND 2 : Outport  Port=3
  AND 3 : Outport  Port=4
  AND 4 : Outport  Port=5
  AND 5 : Outport  Port=6
  AND 6 : Outport  Port=7
  AND 7 : Outport  Port=8
  AND 8 : Outport  Port=9
  OR 0 : Outport  Port=10
  OR 1 : Outport  Port=11
  OR 2 : Outport  Port=12
  OR 3 : Outport  Port=13
  OR 4 : Outport  Port=14
  OR 5 : Outport  Port=15
  OR 6 : Outport  Port=16
  OR 7 : Outport  Port=17
  OR 8 : Outport  Port=18
  wires:
  32b/1 -> b0/1, b1/1, b2/1, b3/1, b4/1, b5/1, b6/1, b7/1, b16/1, b17/1, b18/1, b19/1, b20/1, b21/1, b22/1, b23/1, b24/1, b8/1
  b0/1 -> bool2/1
  b1/1 -> bool1/1
  b2/1 -> bool3/1
  b3/1 -> bool4/1
  b4/1 -> bool5/1
  b5/1 -> bool6/1
  b6/1 -> bool7/1
  b7/1 -> bool8/1
  b16/1 -> bool9/1
  b17/1 -> bool10/1
  b18/1 -> bool11/1
  b19/1 -> bool12/1
  b20/1 -> bool13/1
  b21/1 -> bool14/1
  b22/1 -> bool15/1
  b23/1 -> bool16/1
  bool2/1 -> AND 0/1
  bool1/1 -> AND 1/1
  bool3/1 -> AND 2/1
  bool4/1 -> AND 3/1
  bool5/1 -> AND 4/1
  bool6/1 -> AND 5/1
  bool7/1 -> AND 6/1
  bool8/1 -> AND 7/1
  bool9/1 -> OR 0/1
  bool10/1 -> OR 1/1
  bool11/1 -> OR 2/1
  bool12/1 -> OR 3/1
  bool13/1 -> OR 4/1
  bool14/1 -> OR 5/1
  bool15/1 -> OR 6/1
  bool16/1 -> OR 7/1
  b8/1 -> bool17/1
  bool17/1 -> AND 8/1
  b24/1 -> bool18/1
  bool18/1 -> OR 8/1

== system w2_warplab_trigger_proc/Registers/Output Configuration Slice15 ==
  32b : Inport
  (LSB+0):(LSB+4) : xbsIndex_r4/Slice  nbits=5  boolean_output=off  mode=Lower Bit Location + Width  bit1=0  base1=MSB of Input  bit0=0  base0=LSB of Input  dbl_ovrd=off  block_type=slice
  b31 : xbsIndex_r4/Slice  nbits=1  boolean_output=off  mode=Lower Bit Location + Width  bit1=0  base1=MSB of Input  bit0=31  base0=LSB of Input  dbl_ovrd=off  block_type=slice
  bool17 : xbsIndex_r4/Convert  gui_display_data_type=Boolean  arith_type=Boolean  n_bits=16  bin_pt=14  float_type=Single  exp_bits=8  fraction_bits=24  quantization=Truncate  overflow=Wrap  en=off  latency=0  dbl_ovrd=off  pipeline=off  block_type=convert
  DLY : Outport
  RESET : Outport  Port=2
  wires:
  32b/1 -> b31/1, (LSB+0):(LSB+4)/1
  b31/1 -> bool17/1
  bool17/1 -> RESET/1
  (LSB+0):(LSB+4)/1 -> DLY/1

== system w2_warplab_trigger_proc/Registers/Output Configuration Slice16 ==
  32b : Inport
  b0 : xbsIndex_r4/Slice  nbits=1  boolean_output=off  mode=Lower Bit Location + Width  bit1=0  base1=MSB of Input  bit0=0  base0=LSB of Input  dbl_ovrd=off  block_type=slice
  b1 : xbsIndex_r4/Slice  nbits=1  boolean_output=off  mode=Lower Bit Location + Width  bit1=0  base1=MSB of Input  bit0=1  base0=LSB of Input  dbl_ovrd=off  block_type=slice
  b16 : xbsIndex_r4/Slice  nbits=1  boolean_output=off  mode=Lower Bit Location + Width  bit1=0  base1=MSB of Input  bit0=16  base0=LSB of Input  dbl_ovrd=off  block_type=slice
  b17 : xbsIndex_r4/Slice  nbits=1  boolean_output=off  mode=Lower Bit Location + Width  bit1=0  base1=MSB of Input  bit0=17  base0=LSB of Input  dbl_ovrd=off  block_type=slice
  b18 : xbsIndex_r4/Slice  nbits=1  boolean_output=off  mode=Lower Bit Location + Width  bit1=0  base1=MSB of Input  bit0=18  base0=LSB of Input  dbl_ovrd=off  block_type=slice
  b19 : xbsIndex_r4/Slice  nbits=1  boolean_output=off  mode=Lower Bit Location + Width  bit1=0  base1=MSB of Input  bit0=19  base0=LSB of Input  dbl_ovrd=off  block_type=slice
  b2 : xbsIndex_r4/Slice  nbits=1  boolean_output=off  mode=Lower Bit Location + Width  bit1=0  base1=MSB of Input  bit0=2  base0=LSB of Input  dbl_ovrd=off  block_type=slice
  b20 : xbsIndex_r4/Slice  nbits=1  boolean_output=off  mode=Lower Bit Location + Width  bit1=0  base1=MSB of Input  bit0=20  base0=LSB of Input  dbl_ovrd=off  block_type=slice
  b21 : xbsIndex_r4/Slice  nbits=1  boolean_output=off  mode=Lower Bit Location + Width  bit1=0  base1=MSB of Input  bit0=21  base0=LSB of Input  dbl_ovrd=off  block_type=slice
  b22 : xbsIndex_r4/Slice  nbits=1  boolean_output=off  mode=Lower Bit Location + Width  bit1=0  base1=MSB of Input  bit0=22  base0=LSB of Input  dbl_ovrd=off  block_type=slice
  b23 : xbsIndex_r4/Slice  nbits=1  boolean_output=off  mode=Lower Bit Location + Width  bit1=0  base1=MSB of Input  bit0=23  base0=LSB of Input  dbl_ovrd=off  block_type=slice
  b24 : xbsIndex_r4/Slice  nbits=1  boolean_output=off  mode=Lower Bit Location + Width  bit1=0  base1=MSB of Input  bit0=24  base0=LSB of Input  dbl_ovrd=off  block_type=slice
  b3 : xbsIndex_r4/Slice  nbits=1  boolean_output=off  mode=Lower Bit Location + Width  bit1=0  base1=MSB of Input  bit0=3  base0=LSB of Input  dbl_ovrd=off  block_type=slice
  b4 : xbsIndex_r4/Slice  nbits=1  boolean_output=off  mode=Lower Bit Location + Width  bit1=0  base1=MSB of Input  bit0=4  base0=LSB of Input  dbl_ovrd=off  block_type=slice
  b5 : xbsIndex_r4/Slice  nbits=1  boolean_output=off  mode=Lower Bit Location + Width  bit1=0  base1=MSB of Input  bit0=5  base0=LSB of Input  dbl_ovrd=off  block_type=slice
  b6 : xbsIndex_r4/Slice  nbits=1  boolean_output=off  mode=Lower Bit Location + Width  bit1=0  base1=MSB of Input  bit0=6  base0=LSB of Input  dbl_ovrd=off  block_type=slice
  b7 : xbsIndex_r4/Slice  nbits=1  boolean_output=off  mode=Lower Bit Location + Width  bit1=0  base1=MSB of Input  bit0=7  base0=LSB of Input  dbl_ovrd=off  block_type=slice
  b8 : xbsIndex_r4/Slice  nbits=1  boolean_output=off  mode=Lower Bit Location + Width  bit1=0  base1=MSB of Input  bit0=8  base0=LSB of Input  dbl_ovrd=off  block_type=slice
  bool{1..18} (18 alike) : xbsIndex_r4/Convert  gui_display_data_type=Boolean  arith_type=Boolean  n_bits=16  bin_pt=14  float_type=Single  exp_bits=8  fraction_bits=24  quantization=Truncate  overflow=Wrap  en=off  latency=0  dbl_ovrd=off  pipeline=off  block_type=convert
  AND 0 : Outport
  AND 1 : Outport  Port=2
  AND 2 : Outport  Port=3
  AND 3 : Outport  Port=4
  AND 4 : Outport  Port=5
  AND 5 : Outport  Port=6
  AND 6 : Outport  Port=7
  AND 7 : Outport  Port=8
  AND 8 : Outport  Port=9
  OR 0 : Outport  Port=10
  OR 1 : Outport  Port=11
  OR 2 : Outport  Port=12
  OR 3 : Outport  Port=13
  OR 4 : Outport  Port=14
  OR 5 : Outport  Port=15
  OR 6 : Outport  Port=16
  OR 7 : Outport  Port=17
  OR 8 : Outport  Port=18
  wires:
  32b/1 -> b0/1, b1/1, b2/1, b3/1, b4/1, b5/1, b6/1, b7/1, b16/1, b17/1, b18/1, b19/1, b20/1, b21/1, b22/1, b23/1, b24/1, b8/1
  b0/1 -> bool2/1
  b1/1 -> bool1/1
  b2/1 -> bool3/1
  b3/1 -> bool4/1
  b4/1 -> bool5/1
  b5/1 -> bool6/1
  b6/1 -> bool7/1
  b7/1 -> bool8/1
  b16/1 -> bool9/1
  b17/1 -> bool10/1
  b18/1 -> bool11/1
  b19/1 -> bool12/1
  b20/1 -> bool13/1
  b21/1 -> bool14/1
  b22/1 -> bool15/1
  b23/1 -> bool16/1
  bool2/1 -> AND 0/1
  bool1/1 -> AND 1/1
  bool3/1 -> AND 2/1
  bool4/1 -> AND 3/1
  bool5/1 -> AND 4/1
  bool6/1 -> AND 5/1
  bool7/1 -> AND 6/1
  bool8/1 -> AND 7/1
  bool9/1 -> OR 0/1
  bool10/1 -> OR 1/1
  bool11/1 -> OR 2/1
  bool12/1 -> OR 3/1
  bool13/1 -> OR 4/1
  bool14/1 -> OR 5/1
  bool15/1 -> OR 6/1
  bool16/1 -> OR 7/1
  b8/1 -> bool17/1
  bool17/1 -> AND 8/1
  b24/1 -> bool18/1
  bool18/1 -> OR 8/1

== system w2_warplab_trigger_proc/Registers/Output Configuration Slice7 ==
  32b : Inport
  b0 : xbsIndex_r4/Slice  nbits=1  boolean_output=off  mode=Lower Bit Location + Width  bit1=0  base1=MSB of Input  bit0=0  base0=LSB of Input  dbl_ovrd=off  block_type=slice
  b1 : xbsIndex_r4/Slice  nbits=1  boolean_output=off  mode=Lower Bit Location + Width  bit1=0  base1=MSB of Input  bit0=1  base0=LSB of Input  dbl_ovrd=off  block_type=slice
  b16 : xbsIndex_r4/Slice  nbits=1  boolean_output=off  mode=Lower Bit Location + Width  bit1=0  base1=MSB of Input  bit0=16  base0=LSB of Input  dbl_ovrd=off  block_type=slice
  b17 : xbsIndex_r4/Slice  nbits=1  boolean_output=off  mode=Lower Bit Location + Width  bit1=0  base1=MSB of Input  bit0=17  base0=LSB of Input  dbl_ovrd=off  block_type=slice
  b18 : xbsIndex_r4/Slice  nbits=1  boolean_output=off  mode=Lower Bit Location + Width  bit1=0  base1=MSB of Input  bit0=18  base0=LSB of Input  dbl_ovrd=off  block_type=slice
  b19 : xbsIndex_r4/Slice  nbits=1  boolean_output=off  mode=Lower Bit Location + Width  bit1=0  base1=MSB of Input  bit0=19  base0=LSB of Input  dbl_ovrd=off  block_type=slice
  b2 : xbsIndex_r4/Slice  nbits=1  boolean_output=off  mode=Lower Bit Location + Width  bit1=0  base1=MSB of Input  bit0=2  base0=LSB of Input  dbl_ovrd=off  block_type=slice
  b20 : xbsIndex_r4/Slice  nbits=1  boolean_output=off  mode=Lower Bit Location + Width  bit1=0  base1=MSB of Input  bit0=20  base0=LSB of Input  dbl_ovrd=off  block_type=slice
  b21 : xbsIndex_r4/Slice  nbits=1  boolean_output=off  mode=Lower Bit Location + Width  bit1=0  base1=MSB of Input  bit0=21  base0=LSB of Input  dbl_ovrd=off  block_type=slice
  b22 : xbsIndex_r4/Slice  nbits=1  boolean_output=off  mode=Lower Bit Location + Width  bit1=0  base1=MSB of Input  bit0=22  base0=LSB of Input  dbl_ovrd=off  block_type=slice
  b23 : xbsIndex_r4/Slice  nbits=1  boolean_output=off  mode=Lower Bit Location + Width  bit1=0  base1=MSB of Input  bit0=23  base0=LSB of Input  dbl_ovrd=off  block_type=slice
  b24 : xbsIndex_r4/Slice  nbits=1  boolean_output=off  mode=Lower Bit Location + Width  bit1=0  base1=MSB of Input  bit0=24  base0=LSB of Input  dbl_ovrd=off  block_type=slice
  b3 : xbsIndex_r4/Slice  nbits=1  boolean_output=off  mode=Lower Bit Location + Width  bit1=0  base1=MSB of Input  bit0=3  base0=LSB of Input  dbl_ovrd=off  block_type=slice
  b4 : xbsIndex_r4/Slice  nbits=1  boolean_output=off  mode=Lower Bit Location + Width  bit1=0  base1=MSB of Input  bit0=4  base0=LSB of Input  dbl_ovrd=off  block_type=slice
  b5 : xbsIndex_r4/Slice  nbits=1  boolean_output=off  mode=Lower Bit Location + Width  bit1=0  base1=MSB of Input  bit0=5  base0=LSB of Input  dbl_ovrd=off  block_type=slice
  b6 : xbsIndex_r4/Slice  nbits=1  boolean_output=off  mode=Lower Bit Location + Width  bit1=0  base1=MSB of Input  bit0=6  base0=LSB of Input  dbl_ovrd=off  block_type=slice
  b7 : xbsIndex_r4/Slice  nbits=1  boolean_output=off  mode=Lower Bit Location + Width  bit1=0  base1=MSB of Input  bit0=7  base0=LSB of Input  dbl_ovrd=off  block_type=slice
  b8 : xbsIndex_r4/Slice  nbits=1  boolean_output=off  mode=Lower Bit Location + Width  bit1=0  base1=MSB of Input  bit0=8  base0=LSB of Input  dbl_ovrd=off  block_type=slice
  bool{1..18} (18 alike) : xbsIndex_r4/Convert  gui_display_data_type=Boolean  arith_type=Boolean  n_bits=16  bin_pt=14  float_type=Single  exp_bits=8  fraction_bits=24  quantization=Truncate  overflow=Wrap  en=off  latency=0  dbl_ovrd=off  pipeline=off  block_type=convert
  AND 0 : Outport
  AND 1 : Outport  Port=2
  AND 2 : Outport  Port=3
  AND 3 : Outport  Port=4
  AND 4 : Outport  Port=5
  AND 5 : Outport  Port=6
  AND 6 : Outport  Port=7
  AND 7 : Outport  Port=8
  AND 8 : Outport  Port=9
  OR 0 : Outport  Port=10
  OR 1 : Outport  Port=11
  OR 2 : Outport  Port=12
  OR 3 : Outport  Port=13
  OR 4 : Outport  Port=14
  OR 5 : Outport  Port=15
  OR 6 : Outport  Port=16
  OR 7 : Outport  Port=17
  OR 8 : Outport  Port=18
  wires:
  32b/1 -> b0/1, b1/1, b2/1, b3/1, b4/1, b5/1, b6/1, b7/1, b16/1, b17/1, b18/1, b19/1, b20/1, b21/1, b22/1, b23/1, b24/1, b8/1
  b0/1 -> bool2/1
  b1/1 -> bool1/1
  b2/1 -> bool3/1
  b3/1 -> bool4/1
  b4/1 -> bool5/1
  b5/1 -> bool6/1
  b6/1 -> bool7/1
  b7/1 -> bool8/1
  b16/1 -> bool9/1
  b17/1 -> bool10/1
  b18/1 -> bool11/1
  b19/1 -> bool12/1
  b20/1 -> bool13/1
  b21/1 -> bool14/1
  b22/1 -> bool15/1
  b23/1 -> bool16/1
  bool2/1 -> AND 0/1
  bool1/1 -> AND 1/1
  bool3/1 -> AND 2/1
  bool4/1 -> AND 3/1
  bool5/1 -> AND 4/1
  bool6/1 -> AND 5/1
  bool7/1 -> AND 6/1
  bool8/1 -> AND 7/1
  bool9/1 -> OR 0/1
  bool10/1 -> OR 1/1
  bool11/1 -> OR 2/1
  bool12/1 -> OR 3/1
  bool13/1 -> OR 4/1
  bool14/1 -> OR 5/1
  bool15/1 -> OR 6/1
  bool16/1 -> OR 7/1
  b8/1 -> bool17/1
  bool17/1 -> AND 8/1
  b24/1 -> bool18/1
  bool18/1 -> OR 8/1

== system w2_warplab_trigger_proc/Registers/Output Configuration Slice8 ==
  32b : Inport
  b31 : xbsIndex_r4/Slice  nbits=1  boolean_output=off  mode=Lower Bit Location + Width  bit1=0  base1=MSB of Input  bit0=31  base0=LSB of Input  dbl_ovrd=off  block_type=slice
  b[0:15] : xbsIndex_r4/Slice  nbits=16  boolean_output=off  mode=Lower Bit Location + Width  bit1=0  base1=MSB of Input  bit0=0  base0=LSB of Input  dbl_ovrd=off  block_type=slice
  bool17 : xbsIndex_r4/Convert  gui_display_data_type=Boolean  arith_type=Boolean  n_bits=16  bin_pt=14  float_type=Single  exp_bits=8  fraction_bits=24  quantization=Truncate  overflow=Wrap  en=off  latency=0  dbl_ovrd=off  pipeline=off  block_type=convert
  DLY : Outport
  RESET : Outport  Port=2
  wires:
  32b/1 -> b31/1, b[0:15]/1
  b31/1 -> bool17/1
  bool17/1 -> RESET/1
  b[0:15]/1 -> DLY/1
